simulink model "ss_exercises"  (R2022b)
settings: Solver=VariableStepAuto  StartTime=0.0  StopTime=5  RelTol=1e-3
undefined symbols (not defined in the file): B, C, J, Kt, L, R
settings Model: Creator=Zonularity  LastModifiedBy=Zonularity

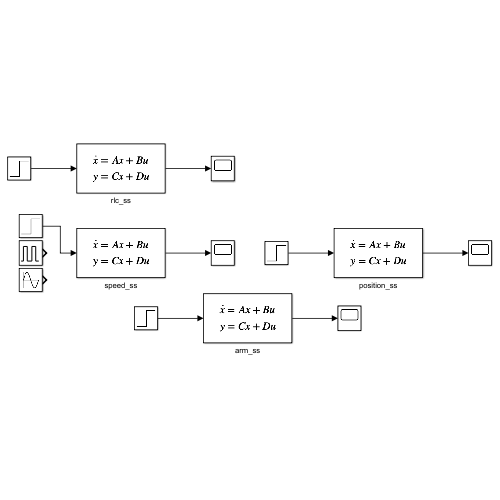
[thumbnail: Simulink's stored preview of the top-level diagram]
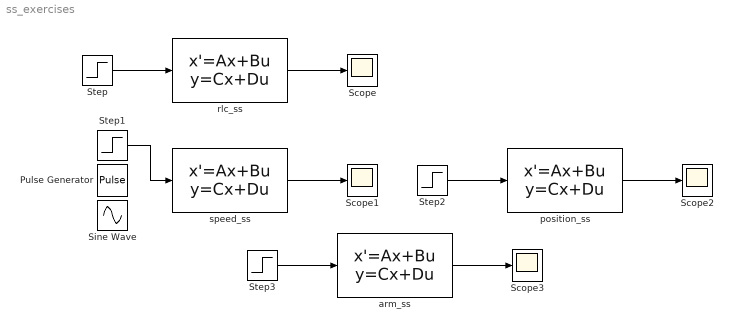
== system ss_exercises ==
  Pulse Generator : DiscretePulseGenerator  PulseType=Time based  Period=1  PulseWidth=50
  Scope{,1..3} (4 alike) : Scope
  Sine Wave : Sin  SampleTime=0
  Step{,1..3} (4 alike) : Step  SampleTime=0
  arm_ss : StateSpace  A=[-1.193e+04 1.951 -113.2 0; 64 0 0 0; 0 128 0 0; 0 0 1 0]  B=[0.25; 0; 0; 0]  C=[0 -0.4713 0 0]  D=0  InitialCondition=0
  position_ss : StateSpace  A=[-1.193e+04 1.951 113.2 0; 64 0 0 0; 0 128 0 0; 0 0 1 0]  B=[8; 0; 0; 0]  C=[0 8.57 0 -0.01379]  InitialCondition=0
  rlc_ss : StateSpace  InitFcn=|  A=[-R/L -1/L; 1/C 0]  B=[1/L; 0]  C=[-R -1]  InitialCondition=0
      | R = 1;
      | L = 1e-3;
      | C = 1e-6;
  speed_ss : StateSpace  InitFcn=|  A=[-B/J, Kt/J; 0, -1/R/L];  B=[0; 1/L];  C=[1, 0]  D=0  InitialCondition=0
      | J = 0.01; % moment of inertia
      | B = 0.001; % friction coefficient
      | Kt = 0.01; % torque constant
      | R = 1; % resistance
      | L = 0.01; % inductance
  wires:
  Step/1 -> rlc_ss/1
  speed_ss/1 -> Scope1/1
  rlc_ss/1 -> Scope/1
  position_ss/1 -> Scope2/1
  arm_ss/1 -> Scope3/1
  Step2/1 -> position_ss/1
  Step3/1 -> arm_ss/1
  Step1/1 -> speed_ss/1
